simulink library "libbha_control_pressure"  (R2015b)
settings: Solver=FixedStepDiscrete  StartTime=0.0  StopTime=Inf  FixedStep=0.004  RelTol=1e-3
PostLoadFcn:
  | , if any(exist('dsrtsu_mdlpostloadfcn', 'file') == [2, 3, 6]), try dsrtsu_mdlpostloadfcn('Execute', bdroot); catch fprintf('Error in PostLoadFcn (dsrtsu_mdlpostloadfcn) for model "%s":\n %s\n', bdroot, lasterr); end, end,
undefined symbols (not defined in the file or in its folder): den, DiscIntNeverNeededParam, num, p1i
undefined symbols (not defined in the file): tA
libraries: libbha_parts_bellows x8, libc_parts_valves x4, simulink x3, libc_parts_tubes x2, libc_control_pressure x1, libbha_parameters x1
settings Model: DSRTSU_INTERNAL_RTI_VER=470  DSRTSU_INTERNAL_RTI_TYPE=rti1007  DSRTSU_INTERNAL_RTIFPGA=60  Creator=Falkenhahn  LastModifiedBy=fav
settings DataIOCC: SaveFormat=Array
settings OptimizationCC: BlockReduction=off  OptimizeBlockIOStorage=off  BufferReuse=off  GlobalBufferReuse=off  ExpressionFolding=off  LocalBlockOutputs=off
settings DebuggingCC: UnderspecifiedInitializationDetection=Classic  MergeDetectMultiDrivingBlocksExec=none  SolverPrmCheckMsg=warning
settings HardwareCC: ProdBitPerPointer=32  ProdLargestAtomicFloat=None  ProdEndianess=BigEndian  ProdWordSize=32  ProdHWDeviceType=Generic->Custom  TargetIntDivRoundTo=Zero  TargetEndianess=BigEndian  TargetHWDeviceType=Generic->Custom
settings RTWCC: SystemTargetFile=rti1007.tlc  MakeCommand=make_rti  TemplateMakefile=rti1007.tmf  Description=dSPACE DS1007 Hardware Platform
settings STFCustomTargetCC: ParMdlRefBuildCompliant=on  ConcurrentExecutionCompliant=off  MatFileLogging=on  SystemTargetFile=rti1007.tlc
settings GRTTargetCC: CompOptLevelCompliant=off  ConcurrentExecutionCompliant=off  GeneratePreprocessorConditionals=Disable all  CombineOutputUpdateFcns=off  GRTInterface=on  UseToolchainInfoCompliant=off  ExtModeMexFile=noextcomm
settings ConfigComp: CovModelRefEnable=Off

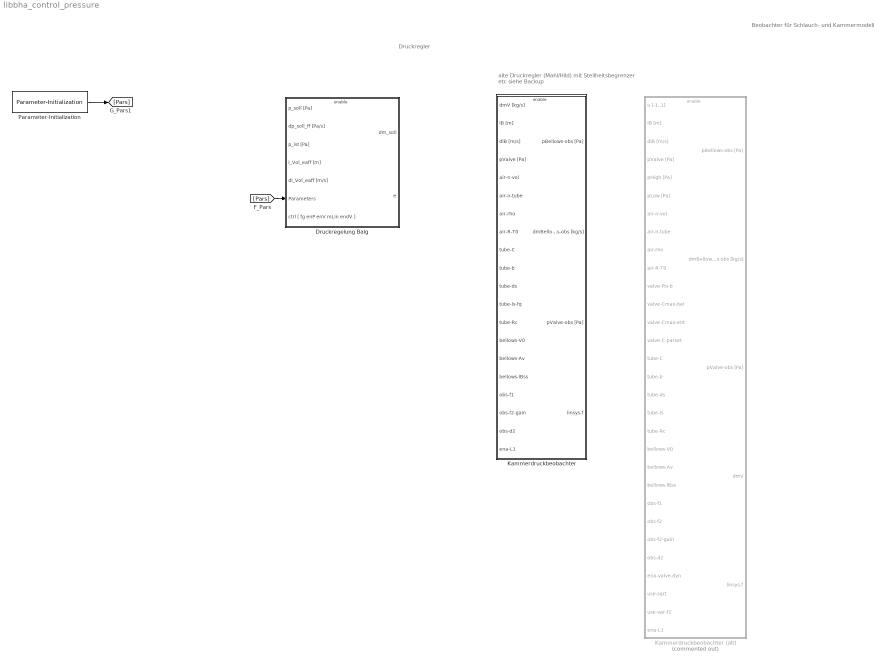
== system libbha_control_pressure ==
  note: alte Druckregler (Mahl/Hild) mit Steilheitsbegrenzer etc
      | siehe Backup
  note: Druckregler
  note: Beobachter für
      | Schlauch- und
      | Kammermodell
  Druckregelung Balg : Subsystem
      settings: AttributesFormatString=|
      | Einzelbalg, Sektion oder Manipulator
      | ohne Schlauchkompensation mit gleichen
      | Parametern und Reglereinstellungen
  Kammerdruckbeobachter : Subsystem
  Kammerdruckbeobachter (alt) : Subsystem  Commented=on
      settings: AttributesFormatString=|
      | neuer Kammerdruckbeobachter
      | ohne Ventilsimulation
      | --> externalisiert
  Parameter-Initialization : libbha_parameters/Parameter-Initialization  bha_var_choice=BHA  tA=CONST.tA
      settings: AttributesFormatString=|
      | BHA-Variable: %<bha_var_choice>
      | sample time: %<tA>
  wires:
  Parameter-Initialization/1 -> [Pars]
  [Pars] -> Druckregelung Balg/6(Parameters)

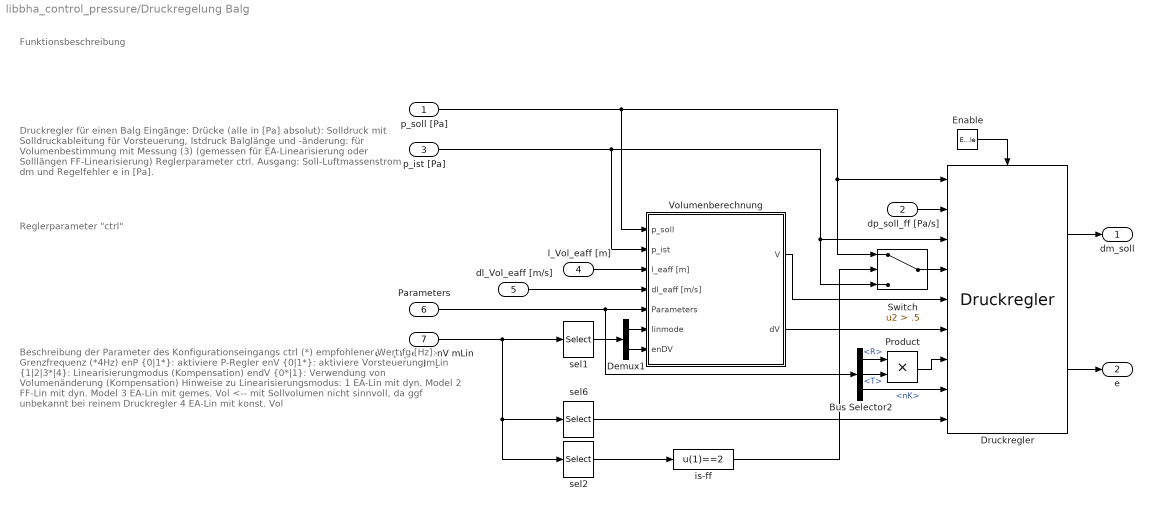
== system libbha_control_pressure/Druckregelung Balg ==
  note: Reglerparameter "ctrl"
  note: Beschreibung der Parameter des Konfigurationseingangs ctrl
      | (*) empfohlener Wert
      |
      | fg [Hz]: Grenzfrequenz (*4Hz)
      | enP {0|1*}: aktiviere P-Regler
      | enV {0|1*}: aktiviere Vorsteuerung
      | mLin {1|2|3*|4}: Linearisierungmodus (Kompensation)
      | endV {0*|1}: Verwendung von Volumenänderung (Kompensation)
      |
      | Hinweise zu Linearisierungsmodus:
      | 1 EA-Lin mit dyn. Model
      | 2 FF-Lin mit dyn. Model
      | 3 EA-Lin mit gemes. Vol  <-- mit Sollvolumen nicht sinnvoll, da ggf unbekannt bei reinem Druckregler
      | 4 EA-Lin mit konst. Vol
  note: Funktionsbeschreibung
  note: Druckregler für einen Balg
      |
      | Eingänge:
      | Drücke (alle in [Pa] absolut): Solldruck mit Solldruckableitung für Vorsteuerung, Istdruck
      | Balglänge und -änderung: für Volumenbestimmung mit Messung (3)
      |     (gemessen für EA-Linearisierung oder Solllängen FF-Linearisierung)
      | Reglerparameter ctrl.
      |
      | Ausgang: Soll-Luftmassenstrom dm und Regelfehler e in [Pa].
  p_soll [Pa] : Inport
  dp_soll_ff [Pa/s] : Inport  Port=2
  p_ist [Pa] : Inport  Port=3
  l_Vol_eaff [m] : Inport  Port=4
  dl_Vol_eaff [m/s] : Inport  Port=5
  Parameters : Inport  Port=6
  ctrl [ fg enP enV mLin endV ] : Inport  Port=7
  Enable : EnablePort  StatesWhenEnabling=reset  ShowOutputPort=on
      settings: AttributesFormatString=%<StatesWhenEnabling> states\nwhen enabling
  Bus Selector2 : BusSelector  OutputSignals=Pressure.R,Pressure.T,Pressure.nK
  Demux1 : Demux  Outputs=2
  Druckregler : libc_control_pressure/Druckregler
  Product : Product
  Switch : Switch  Criteria=u2 > Threshold  Threshold=.5
  Volumenberechnung : Subsystem
  is-ff : Fcn  Expr=u(1)==2
  sel1 : Selector  InputPortWidth=5  IndexOptions=Index vector (dialog)  Indices=[4 5]  OutputSizes=1
  sel2 : Selector  InputPortWidth=5  IndexOptions=Index vector (dialog)  Indices=[4]  OutputSizes=1
  sel6 : Selector  InputPortWidth=5  IndexOptions=Index vector (dialog)  Indices=[1 2 3]  OutputSizes=1
  dm_soll : Outport
  e : Outport  Port=2
  wires:
  ctrl [ fg enP enV mLin endV ]/1 -> sel6/1, sel2/1, sel1/1
  Druckregler/1 -> dm_soll/1
  p_ist [Pa]/1 -> Switch/3, Druckregler/3, Volumenberechnung/2(p_ist)
  dp_soll_ff [Pa/s]/1 -> Druckregler/2
  p_soll [Pa]/1 -> Druckregler/1, Switch/1, Volumenberechnung/1(p_soll)
  l_Vol_eaff [m]/1 -> Volumenberechnung/3(l_eaff [m])
  Demux1/1 -> Volumenberechnung/6(linmode)
  Demux1/2 -> Volumenberechnung/7(enDV)
  sel1/1 -> Demux1/1
  Parameters/1 -> Volumenberechnung/5(Parameters), Bus Selector2/1
  Druckregler/2 -> e/1
  sel2/1 -> is-ff/1
  is-ff/1 -> Switch/2
  sel6/1 -> Druckregler/9
  Bus Selector2/1 -> Product/1  "<R>"
  Bus Selector2/2 -> Product/2  "<T>"
  Bus Selector2/3 -> Druckregler/8  "<nK>"
  Product/1 -> Druckregler/7
  Enable/1 -> Druckregler/Enable
  Volumenberechnung/2(dV) -> Druckregler/6
  Volumenberechnung/1(V) -> Druckregler/5
  dl_Vol_eaff [m/s]/1 -> Volumenberechnung/4(dl_eaff [m/s])
  Switch/1 -> Druckregler/4

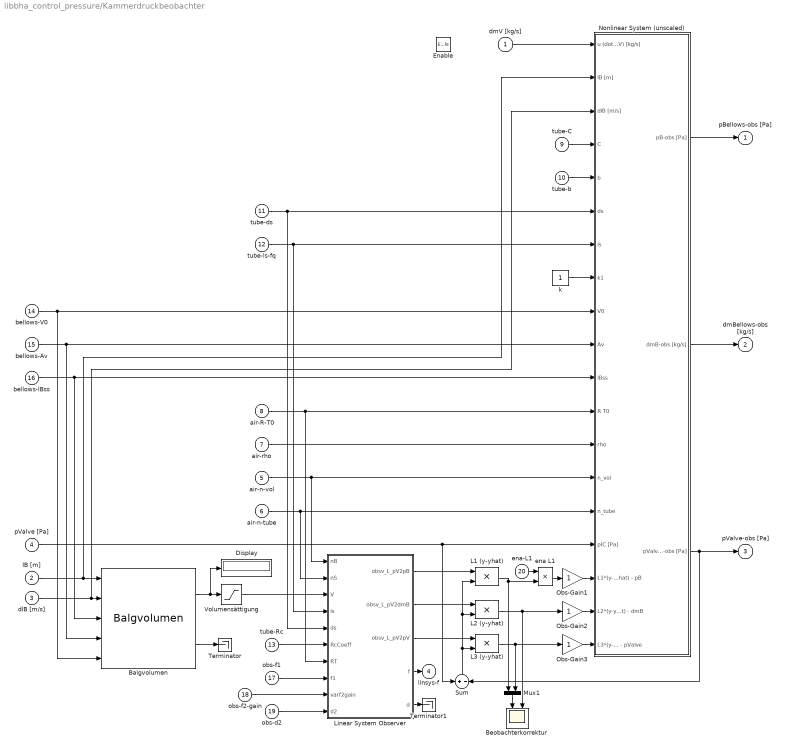
== system libbha_control_pressure/Kammerdruckbeobachter ==
  dmV [kg/s] : Inport
  lB [m] : Inport  Port=2
  dlB [m/s] : Inport  Port=3
  pValve [Pa] : Inport  Port=4
  air-n-vol : Inport  Port=5
  air-n-tube : Inport  Port=6
  air-rho : Inport  Port=7
  air-R-T0 : Inport  Port=8
  tube-C : Inport  Port=9
  tube-b : Inport  Port=10
  tube-ds : Inport  Port=11
  tube-ls-fq : Inport  Port=12
  tube-Rc : Inport  Port=13
  bellows-V0 : Inport  Port=14
  bellows-Av : Inport  Port=15
  bellows-lBss : Inport  Port=16
  obs-f1 : Inport  Port=17
  obs-f2-gain : Inport  Port=18
  obs-d2 : Inport  Port=19
  ena-L1 : Inport  Port=20
  Enable : EnablePort  StatesWhenEnabling=reset
  Balgvolumen : libbha_parts_bellows/Balgvolumen
  Beobachterkorrektur : Scope  NumInputPorts=2
  Display : Display
  L1 (y-yhat) : Product
      settings: AttributesFormatString=sat: 0.1e5
  L2 (y-yhat) : Product
  L3 (y-yhat) : Product
  Linear System Observer : MATLAB Function  TreatAsAtomicUnit=on
      settings: AttributesFormatString=|
      | Lineares System: kein Volumenänderungseinfluss auf Beobachterverstärkung
      | Nichtlin. System (Simulation): Volumen und Volumenänderung in Druckaufbaudynamik
  Mux1 : Mux  Inputs=2
  Nonlinear System (unscaled) : Subsystem
  Obs-Gain1 : Gain
  Obs-Gain2 : Gain
  Obs-Gain3 : Gain
  Sum : Sum  Inputs=+|-
  Terminator : Terminator
  Terminator1 : Terminator
  Volumensättigung : Saturate  UpperLimit=inf  LowerLimit=7e-5
      settings: AttributesFormatString=|
      | min 70 ml
      | ~200 bis 400 ml
  ena L1 : Product
  k : Constant
      settings: AttributesFormatString=nonlinear damping
  pBellows-obs [Pa] : Outport
  dmBellows-obs [kg/s] : Outport  Port=2
  pValve-obs [Pa] : Outport  Port=3
  linsys-f : Outport  Port=4
  wires:
  dmV [kg/s]/1 -> Nonlinear System (unscaled)/1(u (dotmV) [kg/s])
  ena-L1/1 -> ena L1/1
  ena L1/1 -> Obs-Gain1/1
  tube-ds/1 -> Linear System Observer/5(ds), Nonlinear System (unscaled)/6(ds)
  tube-C/1 -> Nonlinear System (unscaled)/4(C)
  L1 (y-yhat)/1 -> Mux1/1, ena L1/2
  Sum/1 -> L2 (y-yhat)/2, L1 (y-yhat)/2, L3 (y-yhat)/2
  Nonlinear System (unscaled)/3(pValve-obs [Pa]) -> Sum/2, pValve-obs [Pa]/1
  Nonlinear System (unscaled)/1(pB-obs [Pa]) -> pBellows-obs [Pa]/1
  Nonlinear System (unscaled)/2(dmB-obs [kg/s]) -> dmBellows-obs [kg/s]/1
  L2 (y-yhat)/1 -> Beobachterkorrektur/2, Obs-Gain2/1
  L3 (y-yhat)/1 -> Mux1/2, Obs-Gain3/1
  Linear System Observer/2(obsv_L_pV2dmB) -> L2 (y-yhat)/1
  Linear System Observer/3(obsv_L_pV2pV) -> L3 (y-yhat)/1
  Linear System Observer/1(obsv_L_pV2pB) -> L1 (y-yhat)/1
  tube-b/1 -> Nonlinear System (unscaled)/5(b)
  lB [m]/1 -> Nonlinear System (unscaled)/2(lB [m]), Balgvolumen/1
  k/1 -> Nonlinear System (unscaled)/8(k1)
  air-n-tube/1 -> Linear System Observer/2(nS), Nonlinear System (unscaled)/15(n_tube)
  bellows-V0/1 -> Balgvolumen/5, Nonlinear System (unscaled)/9(V0)
  bellows-lBss/1 -> Balgvolumen/3, Nonlinear System (unscaled)/11(lBss)
  tube-ls-fq/1 -> Linear System Observer/4(ls), Nonlinear System (unscaled)/7(ls)
  Balgvolumen/1 -> Display/1, Volumensättigung/1
  Balgvolumen/2 -> Terminator/1
  dlB [m/s]/1 -> Nonlinear System (unscaled)/3(dlB [m/s]), Balgvolumen/2
  bellows-Av/1 -> Balgvolumen/4, Nonlinear System (unscaled)/10(Av)
  tube-Rc/1 -> Linear System Observer/6(RcCoeff)
  air-rho/1 -> Nonlinear System (unscaled)/13(rho)
  air-R-T0/1 -> Linear System Observer/7(RT), Nonlinear System (unscaled)/12(R T0)
  obs-f1/1 -> Linear System Observer/8(f1)
  obs-d2/1 -> Linear System Observer/10(d2)
  Linear System Observer/5(d) -> Terminator1/1
  Linear System Observer/4(f) -> linsys-f/1
  air-n-vol/1 -> Linear System Observer/1(nB), Nonlinear System (unscaled)/14(n_vol)
  pValve [Pa]/1 -> Sum/1, Nonlinear System (unscaled)/16(pIC [Pa])
  Mux1/1 -> Beobachterkorrektur/1
  Obs-Gain2/1 -> Nonlinear System (unscaled)/18(L2*(y-yhat) - dmB)
  Obs-Gain3/1 -> Nonlinear System (unscaled)/19(L3*(y-yhat) - pValve)
  Obs-Gain1/1 -> Nonlinear System (unscaled)/17(L1*(y-yhat) - pB)
  obs-f2-gain/1 -> Linear System Observer/9(varf2gain)
  Volumensättigung/1 -> Linear System Observer/3(V)

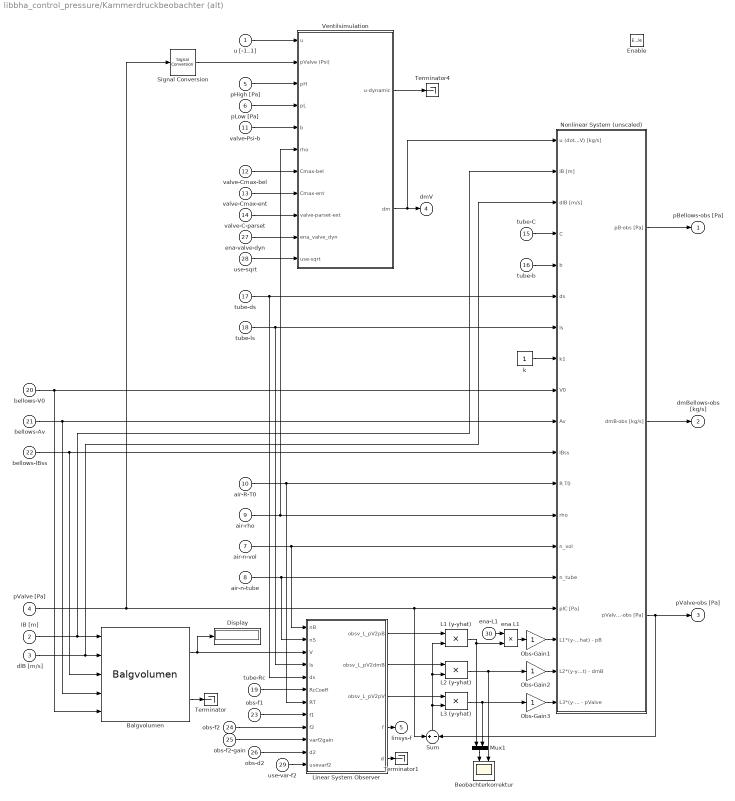
== system libbha_control_pressure/Kammerdruckbeobachter (alt) ==
  u [-1..1] : Inport
  lB [m] : Inport  Port=2
  dlB [m/s] : Inport  Port=3
  pValve [Pa] : Inport  Port=4
  pHigh [Pa] : Inport  Port=5
  pLow [Pa] : Inport  Port=6
  air-n-vol : Inport  Port=7
  air-n-tube : Inport  Port=8
  air-rho : Inport  Port=9
  air-R-T0 : Inport  Port=10
  valve-Psi-b : Inport  Port=11
  valve-Cmax-bel : Inport  Port=12
  valve-Cmax-ent : Inport  Port=13
  valve-C-parset : Inport  Port=14
  tube-C : Inport  Port=15
  tube-b : Inport  Port=16
  tube-ds : Inport  Port=17
  tube-ls : Inport  Port=18
  tube-Rc : Inport  Port=19
  bellows-V0 : Inport  Port=20
  bellows-Av : Inport  Port=21
  bellows-lBss : Inport  Port=22
  obs-f1 : Inport  Port=23
  obs-f2 : Inport  Port=24
  obs-f2-gain : Inport  Port=25
  obs-d2 : Inport  Port=26
  ena-valve-dyn : Inport  Port=27
  use-sqrt : Inport  Port=28
  use-var-f2 : Inport  Port=29
  ena-L1 : Inport  Port=30
  Enable : EnablePort  StatesWhenEnabling=reset
  Balgvolumen : libbha_parts_bellows/Balgvolumen
  Beobachterkorrektur : Scope  NumInputPorts=2
  Display : Display
  L1 (y-yhat) : Product
      settings: AttributesFormatString=sat: 0.1e5
  L2 (y-yhat) : Product
  L3 (y-yhat) : Product
  Linear System Observer : MATLAB Function  TreatAsAtomicUnit=on
      settings: AttributesFormatString=|
      | Lineares System: kein Volumenänderungseinfluss auf Beobachterverstärkung
      | Nichtlin. System (Simulation): Volumen und Volumenänderung in Druckaufbaudynamik
  Mux1 : Mux  Inputs=2
  Nonlinear System (unscaled) : Subsystem
  Obs-Gain1 : Gain
  Obs-Gain2 : Gain
  Obs-Gain3 : Gain
  Signal Conversion : SignalConversion
      settings: AttributesFormatString=|
      | statt des gemessenen
      | Ventildrucks könnte
      | hier auch der beobachtete
      | Ventildruck verwendet
      | werden, aber die zusätzliche
      | Rückführung könnte
      | unerwartete Effekte bringen.
  Sum : Sum  Inputs=+|-
  Terminator : Terminator
  Terminator1 : Terminator
  Terminator4 : Terminator
  Ventilsimulation : Subsystem
  ena L1 : Product
  k : Constant
      settings: AttributesFormatString=nonlinear damping
  pBellows-obs [Pa] : Outport
  dmBellows-obs [kg/s] : Outport  Port=2
  pValve-obs [Pa] : Outport  Port=3
  dmV : Outport  Port=4
  linsys-f : Outport  Port=5
  wires:
  ena-L1/1 -> ena L1/1
  ena L1/1 -> Obs-Gain1/1
  ena-valve-dyn/1 -> Ventilsimulation/10(ena_valve_dyn)
  tube-ds/1 -> Linear System Observer/5(ds), Nonlinear System (unscaled)/6(ds)
  tube-C/1 -> Nonlinear System (unscaled)/4(C)
  L1 (y-yhat)/1 -> Mux1/1, ena L1/2
  Sum/1 -> L2 (y-yhat)/2, L1 (y-yhat)/2, L3 (y-yhat)/2
  Nonlinear System (unscaled)/3(pValve-obs [Pa]) -> Sum/2, pValve-obs [Pa]/1
  Nonlinear System (unscaled)/1(pB-obs [Pa]) -> pBellows-obs [Pa]/1
  Nonlinear System (unscaled)/2(dmB-obs [kg/s]) -> dmBellows-obs [kg/s]/1
  L2 (y-yhat)/1 -> Beobachterkorrektur/2, Obs-Gain2/1
  L3 (y-yhat)/1 -> Mux1/2, Obs-Gain3/1
  Linear System Observer/2(obsv_L_pV2dmB) -> L2 (y-yhat)/1
  Linear System Observer/3(obsv_L_pV2pV) -> L3 (y-yhat)/1
  Linear System Observer/1(obsv_L_pV2pB) -> L1 (y-yhat)/1
  tube-b/1 -> Nonlinear System (unscaled)/5(b)
  lB [m]/1 -> Balgvolumen/1, Nonlinear System (unscaled)/2(lB [m])
  k/1 -> Nonlinear System (unscaled)/8(k1)
  air-n-tube/1 -> Linear System Observer/2(nS), Nonlinear System (unscaled)/15(n_tube)
  bellows-V0/1 -> Balgvolumen/5, Nonlinear System (unscaled)/9(V0)
  bellows-lBss/1 -> Balgvolumen/3, Nonlinear System (unscaled)/11(lBss)
  tube-ls/1 -> Linear System Observer/4(ls), Nonlinear System (unscaled)/7(ls)
  Balgvolumen/1 -> Display/1, Linear System Observer/3(V)
  Balgvolumen/2 -> Terminator/1
  dlB [m/s]/1 -> Balgvolumen/2, Nonlinear System (unscaled)/3(dlB [m/s])
  bellows-Av/1 -> Balgvolumen/4, Nonlinear System (unscaled)/10(Av)
  tube-Rc/1 -> Linear System Observer/6(RcCoeff)
  u [-1..1]/1 -> Ventilsimulation/1(u)
  air-rho/1 -> Nonlinear System (unscaled)/13(rho), Ventilsimulation/6(rho)
  air-R-T0/1 -> Linear System Observer/7(RT), Nonlinear System (unscaled)/12(R T0)
  valve-Cmax-bel/1 -> Ventilsimulation/7(Cmax-bel)
  valve-C-parset/1 -> Ventilsimulation/9(valve-parset-ext)
  pHigh [Pa]/1 -> Ventilsimulation/3(pH)
  pLow [Pa]/1 -> Ventilsimulation/4(pL)
  obs-f1/1 -> Linear System Observer/8(f1)
  obs-d2/1 -> Linear System Observer/11(d2)
  obs-f2/1 -> Linear System Observer/9(f2)
  valve-Psi-b/1 -> Ventilsimulation/5(b)
  Linear System Observer/5(d) -> Terminator1/1
  Linear System Observer/4(f) -> linsys-f/1
  air-n-vol/1 -> Linear System Observer/1(nB), Nonlinear System (unscaled)/14(n_vol)
  pValve [Pa]/1 -> Signal Conversion/1, Sum/1, Nonlinear System (unscaled)/16(pIC [Pa])
  valve-Cmax-ent/1 -> Ventilsimulation/8(Cmax-ent)
  Mux1/1 -> Beobachterkorrektur/1
  Obs-Gain2/1 -> Nonlinear System (unscaled)/18(L2*(y-yhat) - dmB)
  Obs-Gain3/1 -> Nonlinear System (unscaled)/19(L3*(y-yhat) - pValve)
  Obs-Gain1/1 -> Nonlinear System (unscaled)/17(L1*(y-yhat) - pB)
  Ventilsimulation/2(dm) -> dmV/1, Nonlinear System (unscaled)/1(u (dotmV) [kg/s])
  use-sqrt/1 -> Ventilsimulation/11(use-sqrt)
  Ventilsimulation/1(u-dynamic) -> Terminator4/1
  Signal Conversion/1 -> Ventilsimulation/2(pValve (Psi))
  obs-f2-gain/1 -> Linear System Observer/10(varf2gain)
  use-var-f2/1 -> Linear System Observer/12(usevarf2)

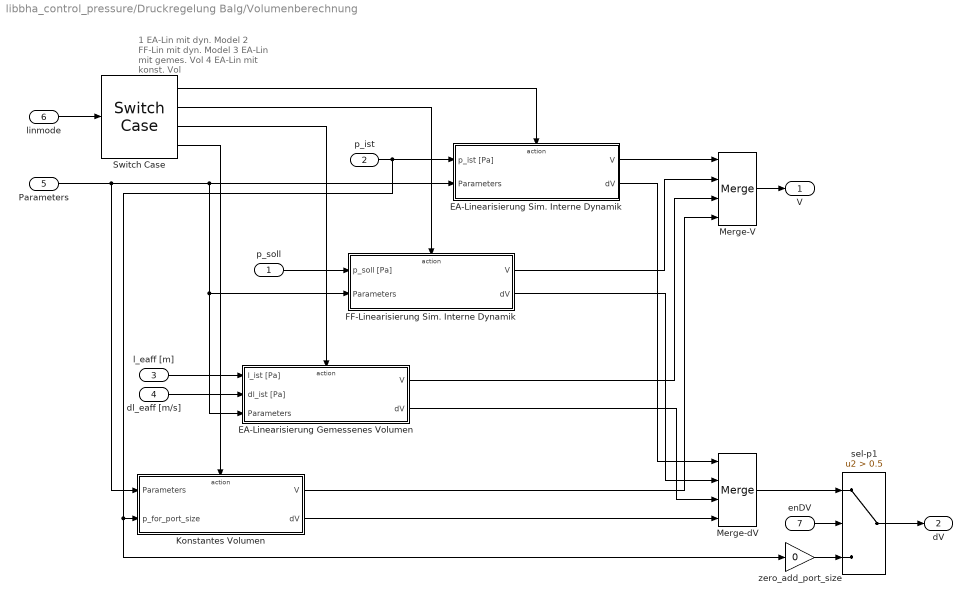
== system libbha_control_pressure/Druckregelung Balg/Volumenberechnung ==
  note: 1 EA-Lin mit dyn. Model
      | 2 FF-Lin mit dyn. Model
      | 3 EA-Lin mit gemes. Vol
      | 4 EA-Lin mit konst. Vol
  p_soll : Inport
  p_ist : Inport  Port=2
  l_eaff [m] : Inport  Port=3
  dl_eaff [m/s] : Inport  Port=4
  Parameters : Inport  Port=5
  linmode : Inport  Port=6
  enDV : Inport  Port=7
  EA-Linearisierung Gemessenes Volumen : Subsystem  TreatAsAtomicUnit=on
  EA-Linearisierung Sim. Interne Dynamik : Subsystem  TreatAsAtomicUnit=on
  FF-Linearisierung Sim. Interne Dynamik : Subsystem  TreatAsAtomicUnit=on
  Konstantes Volumen : Subsystem  TreatAsAtomicUnit=on
  Merge-V : Merge  Inputs=4
  Merge-dV : Merge  Inputs=4
  Switch Case : SwitchCase  CaseConditions={1,2,3}
  sel-p1 : Switch  Criteria=u2 > Threshold  Threshold=0.5
  zero_add_port_size : Gain  Gain=0
  V : Outport
  dV : Outport  Port=2
  wires:
  zero_add_port_size/1 -> sel-p1/3
  enDV/1 -> sel-p1/2
  Merge-V/1 -> V/1
  EA-Linearisierung Sim. Interne Dynamik/1(V) -> Merge-V/1
  EA-Linearisierung Sim. Interne Dynamik/2(dV) -> Merge-dV/1
  FF-Linearisierung Sim. Interne Dynamik/1(V) -> Merge-V/2
  FF-Linearisierung Sim. Interne Dynamik/2(dV) -> Merge-dV/2
  EA-Linearisierung Gemessenes Volumen/1(V) -> Merge-V/3
  EA-Linearisierung Gemessenes Volumen/2(dV) -> Merge-dV/3
  Konstantes Volumen/2(dV) -> Merge-dV/4
  Konstantes Volumen/1(V) -> Merge-V/4
  Merge-dV/1 -> sel-p1/1
  sel-p1/1 -> dV/1
  Switch Case/1 -> EA-Linearisierung Sim. Interne Dynamik/Action
  Switch Case/2 -> FF-Linearisierung Sim. Interne Dynamik/Action
  Switch Case/3 -> EA-Linearisierung Gemessenes Volumen/Action
  Switch Case/4 -> Konstantes Volumen/Action
  Parameters/1 -> Konstantes Volumen/1(Parameters), EA-Linearisierung Gemessenes Volumen/3(Parameters), FF-Linearisierung Sim. Interne Dynamik/2(Parameters), EA-Linearisierung Sim. Interne Dynamik/2(Parameters)
  p_ist/1 -> EA-Linearisierung Sim. Interne Dynamik/1(p_ist [Pa]), Konstantes Volumen/2(p_for_port_size), zero_add_port_size/1
  p_soll/1 -> FF-Linearisierung Sim. Interne Dynamik/1(p_soll [Pa])
  dl_eaff [m/s]/1 -> EA-Linearisierung Gemessenes Volumen/2(dl_ist [Pa])
  l_eaff [m]/1 -> EA-Linearisierung Gemessenes Volumen/1(l_ist [Pa])
  linmode/1 -> Switch Case/1

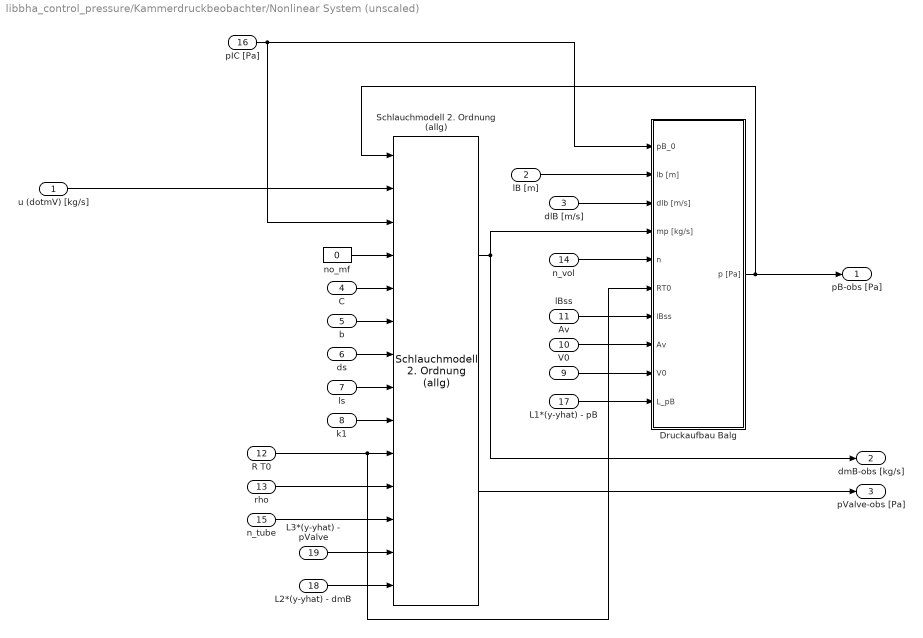
== system libbha_control_pressure/Kammerdruckbeobachter/Nonlinear System (unscaled) ==
  u (dotmV) [kg/s] : Inport
  lB [m] : Inport  Port=2
  dlB [m/s] : Inport  Port=3
  C : Inport  Port=4
  b : Inport  Port=5
  ds : Inport  Port=6
  ls : Inport  Port=7
  k1 : Inport  Port=8
  V0 : Inport  Port=9
  Av : Inport  Port=10
  lBss : Inport  Port=11
  R T0 : Inport  Port=12
  rho : Inport  Port=13
  n_vol : Inport  Port=14
  n_tube : Inport  Port=15
  pIC [Pa] : Inport  Port=16
  L1*(y-yhat) - pB : Inport  Port=17
  L2*(y-yhat) - dmB : Inport  Port=18
  L3*(y-yhat) - pValve : Inport  Port=19
  Druckaufbau Balg : Subsystem
  Schlauchmodell 2. Ordnung (allg) : libc_parts_tubes/Schlauchmodell 2. Ordnung (allg)
  no_mf : Constant  Value=0
  pB-obs [Pa] : Outport
  dmB-obs [kg/s] : Outport  Port=2
  pValve-obs [Pa] : Outport  Port=3
  wires:
  k1/1 -> Schlauchmodell 2. Ordnung (allg)/9
  n_tube/1 -> Schlauchmodell 2. Ordnung (allg)/12
  ls/1 -> Schlauchmodell 2. Ordnung (allg)/8
  ds/1 -> Schlauchmodell 2. Ordnung (allg)/7
  C/1 -> Schlauchmodell 2. Ordnung (allg)/5
  no_mf/1 -> Schlauchmodell 2. Ordnung (allg)/4
  Schlauchmodell 2. Ordnung (allg)/1 -> dmB-obs [kg/s]/1, Druckaufbau Balg/4(mp [kg/s])
  Druckaufbau Balg/1(p [Pa]) -> Schlauchmodell 2. Ordnung (allg)/1, pB-obs [Pa]/1
  Schlauchmodell 2. Ordnung (allg)/2 -> pValve-obs [Pa]/1
  L1*(y-yhat) - pB/1 -> Druckaufbau Balg/10(L_pB)
  L2*(y-yhat) - dmB/1 -> Schlauchmodell 2. Ordnung (allg)/14
  L3*(y-yhat) - pValve/1 -> Schlauchmodell 2. Ordnung (allg)/13
  pIC [Pa]/1 -> Schlauchmodell 2. Ordnung (allg)/3, Druckaufbau Balg/1(pB_0)
  u (dotmV) [kg/s]/1 -> Schlauchmodell 2. Ordnung (allg)/2
  b/1 -> Schlauchmodell 2. Ordnung (allg)/6
  R T0/1 -> Druckaufbau Balg/6(RT0), Schlauchmodell 2. Ordnung (allg)/10
  rho/1 -> Schlauchmodell 2. Ordnung (allg)/11
  lB [m]/1 -> Druckaufbau Balg/2(lb [m])
  V0/1 -> Druckaufbau Balg/9(V0)
  lBss/1 -> Druckaufbau Balg/7(lBss)
  dlB [m/s]/1 -> Druckaufbau Balg/3(dlb [m/s])
  Av/1 -> Druckaufbau Balg/8(Av)
  n_vol/1 -> Druckaufbau Balg/5(n)

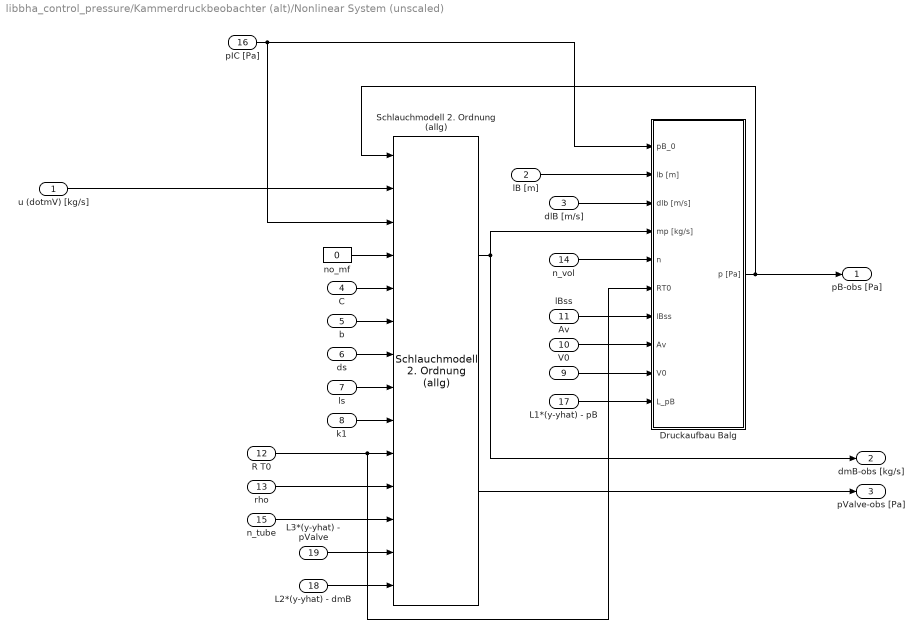
== system libbha_control_pressure/Kammerdruckbeobachter (alt)/Nonlinear System (unscaled) ==
  u (dotmV) [kg/s] : Inport
  lB [m] : Inport  Port=2
  dlB [m/s] : Inport  Port=3
  C : Inport  Port=4
  b : Inport  Port=5
  ds : Inport  Port=6
  ls : Inport  Port=7
  k1 : Inport  Port=8
  V0 : Inport  Port=9
  Av : Inport  Port=10
  lBss : Inport  Port=11
  R T0 : Inport  Port=12
  rho : Inport  Port=13
  n_vol : Inport  Port=14
  n_tube : Inport  Port=15
  pIC [Pa] : Inport  Port=16
  L1*(y-yhat) - pB : Inport  Port=17
  L2*(y-yhat) - dmB : Inport  Port=18
  L3*(y-yhat) - pValve : Inport  Port=19
  Druckaufbau Balg : Subsystem
  Schlauchmodell 2. Ordnung (allg) : libc_parts_tubes/Schlauchmodell 2. Ordnung (allg)
  no_mf : Constant  Value=0
  pB-obs [Pa] : Outport
  dmB-obs [kg/s] : Outport  Port=2
  pValve-obs [Pa] : Outport  Port=3
  wires:
  k1/1 -> Schlauchmodell 2. Ordnung (allg)/9
  n_tube/1 -> Schlauchmodell 2. Ordnung (allg)/12
  ls/1 -> Schlauchmodell 2. Ordnung (allg)/8
  ds/1 -> Schlauchmodell 2. Ordnung (allg)/7
  C/1 -> Schlauchmodell 2. Ordnung (allg)/5
  no_mf/1 -> Schlauchmodell 2. Ordnung (allg)/4
  Schlauchmodell 2. Ordnung (allg)/1 -> dmB-obs [kg/s]/1, Druckaufbau Balg/4(mp [kg/s])
  Druckaufbau Balg/1(p [Pa]) -> Schlauchmodell 2. Ordnung (allg)/1, pB-obs [Pa]/1
  Schlauchmodell 2. Ordnung (allg)/2 -> pValve-obs [Pa]/1
  L1*(y-yhat) - pB/1 -> Druckaufbau Balg/10(L_pB)
  L2*(y-yhat) - dmB/1 -> Schlauchmodell 2. Ordnung (allg)/14
  L3*(y-yhat) - pValve/1 -> Schlauchmodell 2. Ordnung (allg)/13
  pIC [Pa]/1 -> Schlauchmodell 2. Ordnung (allg)/3, Druckaufbau Balg/1(pB_0)
  u (dotmV) [kg/s]/1 -> Schlauchmodell 2. Ordnung (allg)/2
  b/1 -> Schlauchmodell 2. Ordnung (allg)/6
  R T0/1 -> Druckaufbau Balg/6(RT0), Schlauchmodell 2. Ordnung (allg)/10
  rho/1 -> Schlauchmodell 2. Ordnung (allg)/11
  lB [m]/1 -> Druckaufbau Balg/2(lb [m])
  V0/1 -> Druckaufbau Balg/9(V0)
  lBss/1 -> Druckaufbau Balg/7(lBss)
  dlB [m/s]/1 -> Druckaufbau Balg/3(dlb [m/s])
  Av/1 -> Druckaufbau Balg/8(Av)
  n_vol/1 -> Druckaufbau Balg/5(n)

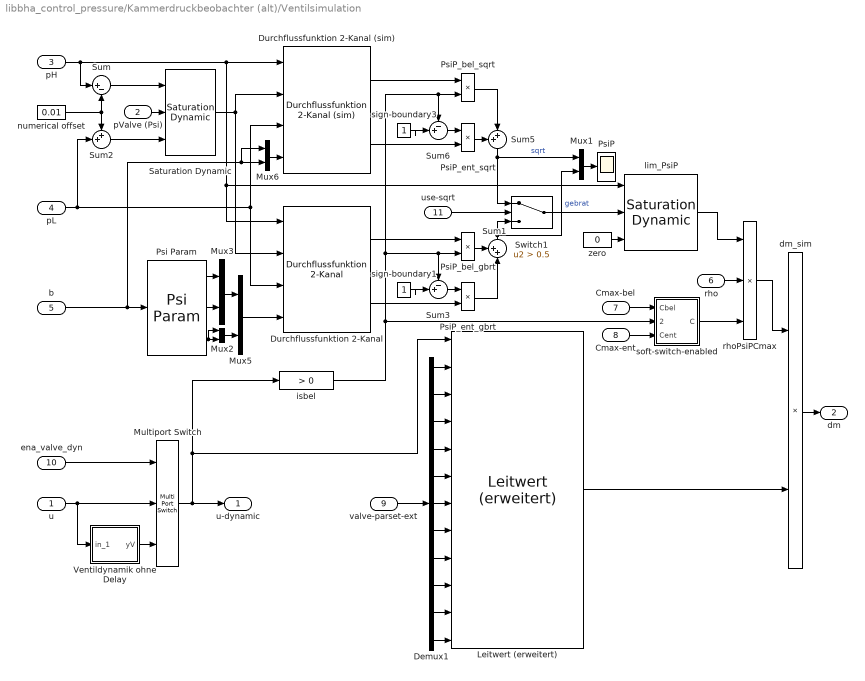
== system libbha_control_pressure/Kammerdruckbeobachter (alt)/Ventilsimulation ==
  u : Inport
  pValve (Psi) : Inport  Port=2
  pH : Inport  Port=3
  pL : Inport  Port=4
  b : Inport  Port=5
  rho : Inport  Port=6
  Cmax-bel : Inport  Port=7
  Cmax-ent : Inport  Port=8
  valve-parset-ext : Inport  Port=9
  ena_valve_dyn : Inport  Port=10
  use-sqrt : Inport  Port=11
  Demux1 : Demux  Outputs=11
  Durchflussfunktion 2-Kanal : libc_parts_valves/Durchflussfunktion 2-Kanal
      settings: AttributesFormatString=gebrochenrational
  Durchflussfunktion 2-Kanal (sim) : libc_parts_valves/Durchflussfunktion 2-Kanal (sim)
      settings: AttributesFormatString=|
      | Wurzelfunktion
      | (nicht geeignet für Ventilinvertierung)
  Leitwert (erweitert) : libc_parts_valves/Leitwert (erweitert)  invertcomp=off
      settings: AttributesFormatString=|
      | inv: Cn --> u (on)
      | hin: u --> Cn (off)
      | Invertiert: %<invertcomp>
  Multiport Switch : MultiPortSwitch  DataPortOrder=Zero-based contiguous  Inputs=2
  Mux{1..3,5..6} (5 alike) : Mux  Inputs=2
  Psi Param : libc_parts_valves/Psi Param
      settings: AttributesFormatString=sqrt -> geb-rat
  PsiP : Scope
  PsiP_bel_gbrt : Product
  PsiP_bel_sqrt : Product
  PsiP_ent_gbrt : Product
  PsiP_ent_sqrt : Product
  Saturation Dynamic : simulink/Discontinuities/Saturation Dynamic  OutMin=[]  OutMax=[]  OutDataTypeStr=Inherit: Same as second input  OutDataType=fixdt(1, 16)  OutScaling=2^-10  DoSatur=off
  Sum : Sum  Inputs=|+-
  Sum1 : Sum  Inputs=++|
  Sum2 : Sum  Inputs=++|
  Sum3 : Sum  Inputs=-+|
  Sum5 : Sum  Inputs=++|
  Sum6 : Sum  Inputs=-+|
  Switch1 : Switch  Criteria=u2 > Threshold  Threshold=0.5
  Ventildynamik ohne Delay : Subsystem  mask(Ventilverzoegerung){wv=200*2*pi, dv=0.6, grenze=0.3, offset=0}
      mask prompts: wv "Eigenfreqenz"; dv "Daempfung"; grenze "Begrenzung"
      mask help: System 2. Ord. mit Begrenzung
      mask init:
      | [num,den]=ord2(wv,dv); t=0:0.5/wv:15/wv; u=0*t+1; u(1)=0;  y=lsim(num,den,u,t);
      mask Display: plot([0:0.1:1],[0 0.05 0.5 0.9 1.0 0.93 0.93 0.97 0.95 0.95 0.95]);
  dm_sim : Product  Inputs=**
  isbel : simulink/Logic and Bit Operations/Compare To Zero  relop=>  OutDataTypeStr=boolean
      settings: AttributesFormatString=|
      | Beim Beobachter macht es keinen Unterschied,
      | ob weicher oder harter Übergang, da u dort
      | immer 0 (klein) ist, jedoch nicht durch 0 dividiert wird
  lim_PsiP : simulink/Discontinuities/Saturation Dynamic  OutMin=[]  OutMax=[]  OutDataTypeStr=Inherit: Same as second input  OutDataType=fixdt(1, 16)  OutScaling=2^-10  DoSatur=off
      settings: AttributesFormatString=|
      | Unterer Schranke
      | im Entlüften nicht
      | pE sondern 0
  numerical offset : Constant  Value=0.01
  rhoPsiPCmax : Product  Inputs=***
  sign-boundary1 : Constant
  sign-boundary3 : Constant
  soft-switch-enabled : MATLAB Function  TreatAsAtomicUnit=on
  zero : Constant  Value=0
  u-dynamic : Outport
  dm : Outport  Port=2
  wires:
  Mux3/1 -> Mux5/1
  Mux2/1 -> Mux5/2
  Psi Param/3 -> Mux2/2, Mux2/1
  Psi Param/2 -> Mux3/2
  Psi Param/1 -> Mux3/1
  Sum5/1 -> Switch1/1, Mux1/1  "sqrt"
  Sum1/1 -> Switch1/3, Mux1/2  "gebrat"
  PsiP_ent_gbrt/1 -> Sum1/2
  PsiP_bel_gbrt/1 -> Sum1/1
  PsiP_ent_sqrt/1 -> Sum5/1
  sign-boundary1/1 -> Sum3/2
  Sum3/1 -> PsiP_ent_gbrt/1
  Durchflussfunktion 2-Kanal/2 -> PsiP_ent_gbrt/2
  Durchflussfunktion 2-Kanal/1 -> PsiP_bel_gbrt/1
  sign-boundary3/1 -> Sum6/2
  Sum6/1 -> PsiP_ent_sqrt/1
  Durchflussfunktion 2-Kanal (sim)/2 -> PsiP_ent_sqrt/2
  Durchflussfunktion 2-Kanal (sim)/1 -> PsiP_bel_sqrt/1
  PsiP_bel_sqrt/1 -> Sum5/2
  Mux6/1 -> Durchflussfunktion 2-Kanal (sim)/4
  Mux5/1 -> Durchflussfunktion 2-Kanal/4
  b/1 -> Psi Param/1, Mux6/2, Mux6/1
  isbel/1 -> soft-switch-enabled/2(alpha), PsiP_bel_sqrt/2, Sum6/1, PsiP_bel_gbrt/2, Sum3/1
  Switch1/1 -> lim_PsiP/2
  Mux1/1 -> PsiP/1
  Demux1/11 -> Leitwert (erweitert)/12
  Demux1/8 -> Leitwert (erweitert)/9
  Demux1/10 -> Leitwert (erweitert)/11
  Demux1/9 -> Leitwert (erweitert)/10
  ena_valve_dyn/1 -> Multiport Switch/1
  zero/1 -> lim_PsiP/3
  Cmax-ent/1 -> soft-switch-enabled/3(Cent)
  soft-switch-enabled/1(C) -> rhoPsiPCmax/3
  Ventildynamik ohne Delay/1(yV) -> Multiport Switch/3
  Cmax-bel/1 -> soft-switch-enabled/1(Cbel)
  rho/1 -> rhoPsiPCmax/2
  pH/1 -> Durchflussfunktion 2-Kanal/1, lim_PsiP/1, Durchflussfunktion 2-Kanal (sim)/1, Sum/1
  Sum/1 -> Saturation Dynamic/1
  lim_PsiP/1 -> rhoPsiPCmax/1
  pValve (Psi)/1 -> Saturation Dynamic/2
  Saturation Dynamic/1 -> Durchflussfunktion 2-Kanal/2, Durchflussfunktion 2-Kanal (sim)/2
  rhoPsiPCmax/1 -> dm_sim/1
  pL/1 -> Durchflussfunktion 2-Kanal/3, Durchflussfunktion 2-Kanal (sim)/3, Sum2/2
  numerical offset/1 -> Sum/2, Sum2/1
  Sum2/1 -> Saturation Dynamic/3
  valve-parset-ext/1 -> Demux1/1
  Multiport Switch/1 -> u-dynamic/1, isbel/1, Leitwert (erweitert)/1
  u/1 -> Ventildynamik ohne Delay/1(in_1), Multiport Switch/2
  Demux1/7 -> Leitwert (erweitert)/8
  Demux1/4 -> Leitwert (erweitert)/5
  Demux1/3 -> Leitwert (erweitert)/4
  Demux1/6 -> Leitwert (erweitert)/7
  Demux1/5 -> Leitwert (erweitert)/6
  Demux1/2 -> Leitwert (erweitert)/3
  Demux1/1 -> Leitwert (erweitert)/2
  Leitwert (erweitert)/1 -> dm_sim/2
  dm_sim/1 -> dm/1
  use-sqrt/1 -> Switch1/2

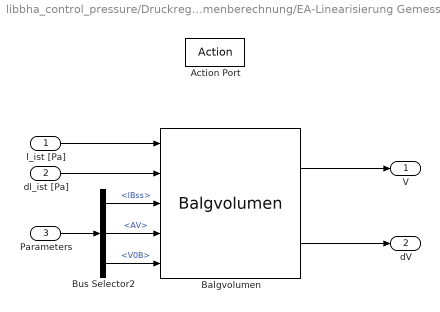
== system libbha_control_pressure/Druckregelung Balg/Volumenberechnung/EA-Linearisierung Gemessenes Volumen ==
  l_ist [Pa] : Inport
  dl_ist [Pa] : Inport  Port=2
  Parameters : Inport  Port=3
  Action Port : ActionPort
  Balgvolumen : libbha_parts_bellows/Balgvolumen
  Bus Selector2 : BusSelector  OutputSignals=Bellows.lBss,Bellows.AV,Bellows.V0B
  V : Outport
  dV : Outport  Port=2
  wires:
  Balgvolumen/1 -> V/1
  Balgvolumen/2 -> dV/1
  l_ist [Pa]/1 -> Balgvolumen/1
  dl_ist [Pa]/1 -> Balgvolumen/2
  Parameters/1 -> Bus Selector2/1
  Bus Selector2/1 -> Balgvolumen/3  "<lBss>"
  Bus Selector2/2 -> Balgvolumen/4  "<AV>"
  Bus Selector2/3 -> Balgvolumen/5  "<V0B>"

== system libbha_control_pressure/Druckregelung Balg/Volumenberechnung/EA-Linearisierung Sim. Interne Dynamik ==
  p_ist [Pa] : Inport
  Parameters : Inport  Port=2
  Action Port : ActionPort
  Interne Dynamik Balgdrucksystem : libbha_parts_bellows/Interne Dynamik Balgdrucksystem
  V : Outport
  dV : Outport  Port=2
  wires:
  p_ist [Pa]/1 -> Interne Dynamik Balgdrucksystem/1
  Parameters/1 -> Interne Dynamik Balgdrucksystem/2
  Interne Dynamik Balgdrucksystem/1 -> V/1
  Interne Dynamik Balgdrucksystem/2 -> dV/1

== system libbha_control_pressure/Druckregelung Balg/Volumenberechnung/FF-Linearisierung Sim. Interne Dynamik ==
  p_soll [Pa] : Inport
  Parameters : Inport  Port=2
  Action Port : ActionPort
  Interne Dynamik Balgdrucksystem : libbha_parts_bellows/Interne Dynamik Balgdrucksystem
  V : Outport
  dV : Outport  Port=2
  wires:
  p_soll [Pa]/1 -> Interne Dynamik Balgdrucksystem/1
  Interne Dynamik Balgdrucksystem/1 -> V/1
  Interne Dynamik Balgdrucksystem/2 -> dV/1
  Parameters/1 -> Interne Dynamik Balgdrucksystem/2

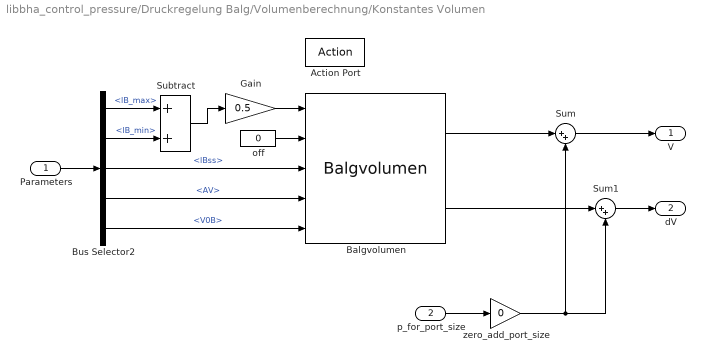
== system libbha_control_pressure/Druckregelung Balg/Volumenberechnung/Konstantes Volumen ==
  Parameters : Inport
  p_for_port_size : Inport  Port=2
  Action Port : ActionPort
  Balgvolumen : libbha_parts_bellows/Balgvolumen
  Bus Selector2 : BusSelector  OutputSignals=Bellows.lB_max,Bellows.lB_min,Bellows.lBss,Bellows.AV,Bellows.V0B
  Gain : Gain  Gain=0.5
  Subtract : Sum
  Sum : Sum  Inputs=|++
  Sum1 : Sum  Inputs=|++
  off : Constant  Value=0
  zero_add_port_size : Gain  Gain=0
  V : Outport
  dV : Outport  Port=2
  wires:
  zero_add_port_size/1 -> Sum/2, Sum1/2
  Sum1/1 -> dV/1
  Sum/1 -> V/1
  p_for_port_size/1 -> zero_add_port_size/1
  off/1 -> Balgvolumen/2
  Parameters/1 -> Bus Selector2/1
  Bus Selector2/3 -> Balgvolumen/3  "<lBss>"
  Bus Selector2/4 -> Balgvolumen/4  "<AV>"
  Bus Selector2/5 -> Balgvolumen/5  "<V0B>"
  Bus Selector2/2 -> Subtract/2  "<lB_min>"
  Bus Selector2/1 -> Subtract/1  "<lB_max>"
  Balgvolumen/2 -> Sum1/1
  Subtract/1 -> Gain/1
  Gain/1 -> Balgvolumen/1
  Balgvolumen/1 -> Sum/1

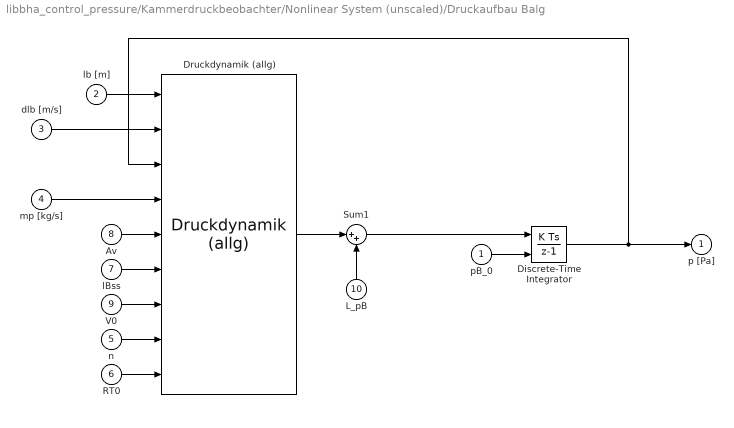
== system libbha_control_pressure/Kammerdruckbeobachter/Nonlinear System (unscaled)/Druckaufbau Balg ==
  pB_0 : Inport
  lb [m] : Inport  Port=2
  dlb [m/s] : Inport  Port=3
  mp [kg/s] : Inport  Port=4
  n : Inport  Port=5
  RT0 : Inport  Port=6
  lBss : Inport  Port=7
  Av : Inport  Port=8
  V0 : Inport  Port=9
  L_pB : Inport  Port=10
  Discrete-Time Integrator : DiscreteIntegrator  InitialConditionSource=external  InitialCondition=p1i  SampleTime=-1  ICPrevOutput=DiscIntNeverNeededParam  ICPrevScaledInput=DiscIntNeverNeededParam
  Druckdynamik (allg) : libbha_parts_bellows/Druckdynamik (allg)
  Sum1 : Sum  Inputs=|++
  p [Pa] : Outport  InitialOutput=0
  wires:
  n/1 -> Druckdynamik (allg)/8
  Druckdynamik (allg)/1 -> Sum1/1
  mp [kg/s]/1 -> Druckdynamik (allg)/4
  Discrete-Time Integrator/1 -> Druckdynamik (allg)/3, p [Pa]/1
  Sum1/1 -> Discrete-Time Integrator/1
  pB_0/1 -> Discrete-Time Integrator/2
  L_pB/1 -> Sum1/2
  dlb [m/s]/1 -> Druckdynamik (allg)/2
  lb [m]/1 -> Druckdynamik (allg)/1
  RT0/1 -> Druckdynamik (allg)/9
  lBss/1 -> Druckdynamik (allg)/6
  Av/1 -> Druckdynamik (allg)/5
  V0/1 -> Druckdynamik (allg)/7

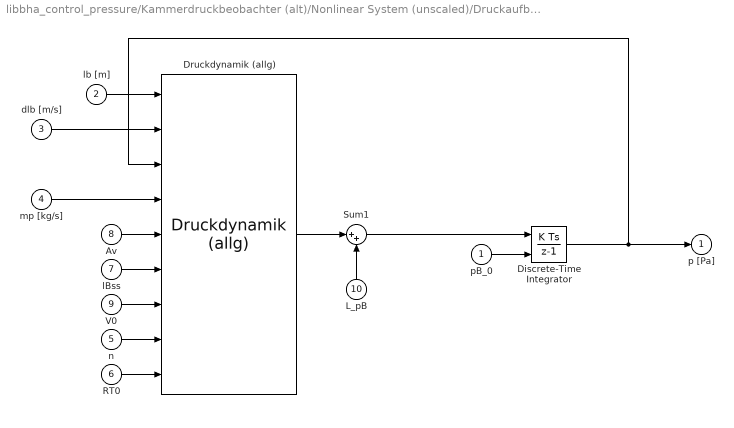
== system libbha_control_pressure/Kammerdruckbeobachter (alt)/Nonlinear System (unscaled)/Druckaufbau Balg ==
  pB_0 : Inport
  lb [m] : Inport  Port=2
  dlb [m/s] : Inport  Port=3
  mp [kg/s] : Inport  Port=4
  n : Inport  Port=5
  RT0 : Inport  Port=6
  lBss : Inport  Port=7
  Av : Inport  Port=8
  V0 : Inport  Port=9
  L_pB : Inport  Port=10
  Discrete-Time Integrator : DiscreteIntegrator  InitialConditionSource=external  InitialCondition=p1i  SampleTime=-1  ICPrevOutput=DiscIntNeverNeededParam  ICPrevScaledInput=DiscIntNeverNeededParam
  Druckdynamik (allg) : libbha_parts_bellows/Druckdynamik (allg)
  Sum1 : Sum  Inputs=|++
  p [Pa] : Outport  InitialOutput=0
  wires:
  n/1 -> Druckdynamik (allg)/8
  Druckdynamik (allg)/1 -> Sum1/1
  mp [kg/s]/1 -> Druckdynamik (allg)/4
  Discrete-Time Integrator/1 -> Druckdynamik (allg)/3, p [Pa]/1
  Sum1/1 -> Discrete-Time Integrator/1
  pB_0/1 -> Discrete-Time Integrator/2
  L_pB/1 -> Sum1/2
  dlb [m/s]/1 -> Druckdynamik (allg)/2
  lb [m]/1 -> Druckdynamik (allg)/1
  RT0/1 -> Druckdynamik (allg)/9
  lBss/1 -> Druckdynamik (allg)/6
  Av/1 -> Druckdynamik (allg)/5
  V0/1 -> Druckdynamik (allg)/7

== system libbha_control_pressure/Kammerdruckbeobachter (alt)/Ventilsimulation/Ventildynamik ohne Delay ==
  in_1 : Inport
  Saturation : Saturate  UpperLimit=grenze  LowerLimit=-grenze
  Sum : Sum  Inputs=+-  SaturateOnIntegerOverflow=on  InputSameDT=on  OutDataTypeStr=Inherit: Same as first input
  Sum2 : Sum  SaturateOnIntegerOverflow=on  InputSameDT=on  OutDataTypeStr=Inherit: Same as first input
  discrete filter : DiscreteTransferFcn  Numerator=num  Denominator=den  SampleTime=TS  mask{wv=wv, dv=dv, TS=tA}
      mask prompts: wv "Grenzfrequenz (rad/s)"; dv "Dämpfung"; TS "Sample Time"
      mask init:
      | csys = tf(wv^2,[1,2*dv*wv,0]);
      | [nums,dens] = tfdata(csys,'v');
      | [num,den] = tfdata(c2d(csys,TS),'v');
      settings: AttributesFormatString=w²/(s² + 2dws)
      mask Display: dpoly(nums,dens)
  p0 : Constant  Value=offset
  yV : Outport  InitialOutput=0
  wires:
  Sum/1 -> Saturation/1
  Saturation/1 -> discrete filter/1
  discrete filter/1 -> Sum/2, Sum2/2
  p0/1 -> Sum2/1
  in_1/1 -> Sum/1
  Sum2/1 -> yV/1

== matlab function libbha_control_pressure/Kammerdruckbeobachter (alt)/Linear System Observer ==
  data: nB input; nS input; V input; ls input; ds input; RcCoeff input; RT input; obsv_L_pV2pB output; f1 input; obsv_L_pV2dmB output; obsv_L_pV2pV output; f2 input; varf2gain input; d2 input; f output; d output; usevarf2 input
function [obsv_L_pV2pB, obsv_L_pV2dmB, obsv_L_pV2pV, f, d] = obsgains(nB, nS, V, ls, ds, RcCoeff, RT, f1, f2, varf2gain, d2, usevarf2)
%#codegen

%% abhängige Systemvariablen
As = (ds/2).^2*pi;
Rc = RcCoeff*8*pi./As.^2; 
    
%% Variablen-Skalierungen
% eigene Volumenskalierung scale_ls, scale_As, scale_V statt Autoskalierung: scale_dm/scale_p (^1 / ^2 / ^3)

scale_dm = 1e3;     % [kg/s]       [kg]->[ g]
scale_p  = 1e-5;    % [kg/m/s²]    [ m]->[nm]
scale_V  = 1e4;     % [m³]         [ m]->[ l] = dm³ statt eigentlich nm³
scale_ls = sqrt(scale_V*scale_p/scale_dm); 
scale_As = sqrt(scale_V*scale_dm/scale_p);
scale_R = scale_p*scale_V/scale_dm;
scale_Rc = scale_p/scale_dm;

nB = nB*1;              % [-]
nS = nS*1;              % [-]
V  = V*scale_V;         % [m³]
RT = RT*scale_R;        % [Pa m³/kg/K = m²/s²/K]
ls = ls*scale_ls;       % [m]
As = As*scale_As;       % [m²]
Rc = Rc*scale_Rc;       % [1/m/s]

%% Analyse
% EV = -w(d+-sqrt(1-d²)   -->   w = sqrt(I²+R²),  d = R/w

ev_real    = -(ls.*Rc)/2; 
ev_imag_sq = ((ls.*Rc).^2)/4 - pi^2/4*nS.*RT./ls.^2 - As./(ls.*V).*nB.*RT;

w = sqrt(ev_real.^2 + abs(ev_imag_sq));
d = -ev_real./w;
f = w/(2*pi);

%% Beobachterberechnung (Ackermann)
% Beobachter-Pole:
% lambda = [-w1; -w2*(d2-sqrt(1-d2^2)*1i); -w2*(d2+sqrt(1-d2^2)*1i)];

if usevarf2 % dynamisch angepasste Sollfrequenzanpassung (abhängig von der Schlauch-Eigenfrequenz)
	f2 = f.*varf2gain;
end

p00 =   (2*pi*f2).^2;
p01 = 2*(2*pi*f2).*d2;

p0 = p00.*(2*pi*f1);
p1 = p01.*(2*pi*f1) + p00;
p2 =      (2*pi*f1) + p01;

% Beobachter Ackermannformel für Ventildruck als Messgröße
% inkl. Rückskalierung von p2dm
obsv_L_pV2pB  =                     4 .* ls .* nS .^ (-1) .* pi .^ (-2) .* RT .^ (-1) .* V .^ (-1) .* (As .* nB .* RT .* ((-1) .* p2 + ls .* Rc) + p0 .* ls .* V);
obsv_L_pV2dmB = scale_p/scale_dm * (As .* ls .^ (-1) .* nS .^ (-1) .* pi .^ (-2) .* RT .^ (-1) .* V .^ (-1) .* (4 .* As .* ls .* nB .* RT + ((-4) .* ls .^ 2 .* (p1 + ls .* Rc .* ((-1) .* p2 + ls .* Rc)) + nS .* pi .^ 2 .* RT) .* V));
obsv_L_pV2pV  =                     p2 + (-1) .* ls .* Rc;

== matlab function libbha_control_pressure/Kammerdruckbeobachter (alt)/Ventilsimulation/soft-switch-enabled ==
  data: Cbel input; C output; alpha input; Cent input
function C = s(Cbel, alpha, Cent)
%#codegen

C = Cbel.*alpha + (1-alpha).*Cent;

== matlab function libbha_control_pressure/Kammerdruckbeobachter/Linear System Observer ==
  data: nB input; nS input; V input; ls input; ds input; RcCoeff input; RT input; obsv_L_pV2pB output; f1 input; obsv_L_pV2dmB output; obsv_L_pV2pV output; varf2gain input; d2 input; f output; d output
%function [obsv_L_pV2pB, obsv_L_pV2dmB, obsv_L_pV2pV, f, d] = obsgains(nB, nS, V, ls, ds, RcCoeff, RT, f1, f2, varf2gain, d2, usevarf2)
function [obsv_L_pV2pB, obsv_L_pV2dmB, obsv_L_pV2pV, f, d] = obsgains(nB, nS, V, ls, ds, RcCoeff, RT, f1, varf2gain, d2)
%#codegen

%% abhängige Systemvariablen
As = (ds/2).^2*pi;
Rc = RcCoeff*8*pi./As.^2; 
    
%% Variablen-Skalierungen
% eigene Volumenskalierung scale_ls, scale_As, scale_V statt Autoskalierung: scale_dm/scale_p (^1 / ^2 / ^3)

scale_dm = 1e3;     % [kg/s]       [kg]->[ g]
scale_p  = 1e-5;    % [kg/m/s²]    [ m]->[nm]
scale_V  = 1e4;     % [m³]         [ m]->[ l] = dm³ statt eigentlich nm³
scale_ls = sqrt(scale_V*scale_p/scale_dm); 
scale_As = sqrt(scale_V*scale_dm/scale_p);
scale_R = scale_p*scale_V/scale_dm;
scale_Rc = scale_p/scale_dm;

nB = nB*1;              % [-]
nS = nS*1;              % [-]
V  = V*scale_V;         % [m³]
RT = RT*scale_R;        % [Pa m³/kg/K = m²/s²/K]
ls = ls*scale_ls;       % [m]
As = As*scale_As;       % [m²]
Rc = Rc*scale_Rc;       % [1/m/s]

%% Analyse
% EV = -w(d+-sqrt(1-d²)   -->   w = sqrt(I²+R²),  d = R/w

ev_real    = -(ls.*Rc)/2; 
ev_imag_sq = ((ls.*Rc).^2)/4 - pi^2/4*nS.*RT./ls.^2 - As./(ls.*V).*nB.*RT;

w = sqrt(ev_real.^2 + abs(ev_imag_sq));
d = -ev_real./w;
f = w/(2*pi);

%% Beobachterberechnung (Ackermann)
% Beobachter-Pole:
% lambda = [-w1; -w2*(d2-sqrt(1-d2^2)*1i); -w2*(d2+sqrt(1-d2^2)*1i)];

%if usevarf2 % dynamisch angepasste Sollfrequenzanpassung (abhängig von der Schlauch-Eigenfrequenz)
	f2 = f.*varf2gain;
%end

p00 =   (2*pi*f2).^2;
p01 = 2*(2*pi*f2).*d2;

p0 = p00.*(2*pi*f1);
p1 = p01.*(2*pi*f1) + p00;
p2 =      (2*pi*f1) + p01;

% Beobachter Ackermannformel für Ventildruck als Messgröße
% inkl. Rückskalierung von p2dm
obsv_L_pV2pB  =                     4 .* ls .* nS .^ (-1) .* pi .^ (-2) .* RT .^ (-1) .* V .^ (-1) .* (As .* nB .* RT .* ((-1) .* p2 + ls .* Rc) + p0 .* ls .* V);
obsv_L_pV2dmB = scale_p/scale_dm * (As .* ls .^ (-1) .* nS .^ (-1) .* pi .^ (-2) .* RT .^ (-1) .* V .^ (-1) .* (4 .* As .* ls .* nB .* RT + ((-4) .* ls .^ 2 .* (p1 + ls .* Rc .* ((-1) .* p2 + ls .* Rc)) + nS .* pi .^ 2 .* RT) .* V));
obsv_L_pV2pV  =                     p2 + (-1) .* ls .* Rc;
